simulink model "FHA_2P4S_Boosted"  (R2018a)
settings: Solver=VariableStepAuto  StartTime=0.0  StopTime=0.01  MaxStep=1e-5  RelTol=1e-3
values from neighbouring files (symbols this model uses):
  fop = 203    [inductance_calculation.m]
  M = 10^6*M    (= 4.12942555049)    [design_code.m]    (also in inductance_calculation.m = [M11 M12; M12' M22])
  R = [R11 R12;R12' R22]    [inductance_calculation.m]
  Vin_peak = 127    [inductance_calculation.m]
libraries: powerlib x49, powerlib_meascontrol x6
settings Model: Creator=user  LastModifiedBy=enes_

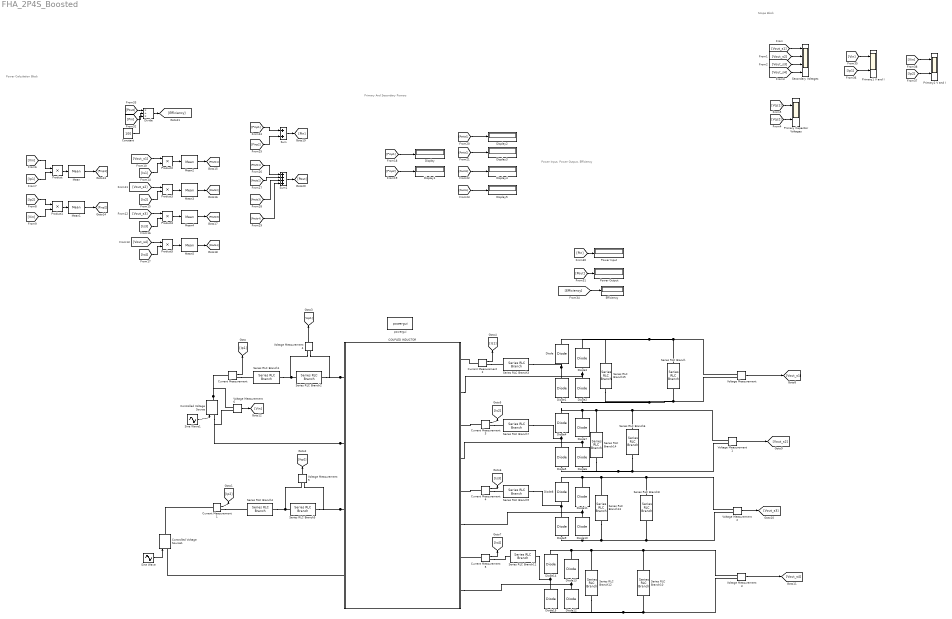
== system FHA_2P4S_Boosted ==
  note: Scope Block
  note: Primary And Secondary Powers
  note: Power Calculation Block
  note: Power Input,
      | Power Output,
      | Efficiency
  COUPLED INDUCTOR : Subsystem
  Constant : Constant  Value=100
  Controlled Voltage Source : powerlib/Electrical Sources/Controlled Voltage Source  Initialize=on  Source_Type=AC  Amplitude=0  Phase=0  Frequency=0  Measurements=None
  Controlled Voltage Source1 : powerlib/Electrical Sources/Controlled Voltage Source  Initialize=on  Source_Type=AC  Amplitude=0  Phase=0  Frequency=0  Measurements=None
  Current Measurement{,1..5} (6 alike) : powerlib/Measurements/Current Measurement  PhasorSimulation=off  OutputType=Complex  PSBequivalent=0
  Diode{,1..15} (16 alike) : powerlib/Power Electronics/Diode  Ron=0.001  Lon=0  Vf=0.8  IC=0  UseSnubber=0  Rs=inf  Cs=250e-9  Measurements=off
  Display{,1..5} (6 alike) : Display
  Divide : Product  Inputs=*/*
  Efficiency : Display
  Mean{,1..5} (6 alike) : powerlib_meascontrol/Measurements/Mean  Freq=fop*1000  Vinit=0  Ts=0
  Power Input : Display
  Power Output : Display
  Primary Capacitor Voltages : Scope  NumInputPorts=2
  Primary1 V and I : Scope  NumInputPorts=2
  Primary2 V and I : Scope  NumInputPorts=2
  Product{,1..5} (6 alike) : Product
  Secondary Voltages : Scope  NumInputPorts=4
  Series RLC Branch{,6,8,10} (4 alike) : powerlib/Elements/Series RLC Branch  LConnTagsString=__new0  RConnTagsString=__new0  BranchType=R  Resistance=15  Inductance=1e-3  SetiL0=off  InitialCurrent=0  Capacitance=1e-6  Setx0=off  InitialVoltage=0  Measurements=None
  Series RLC Branch1 : powerlib/Elements/Series RLC Branch  LConnTagsString=__new0  RConnTagsString=__new0  BranchType=R  Resistance=0.01  Inductance=1e-3  SetiL0=off  InitialCurrent=0  Capacitance=1e-6  Setx0=off  InitialVoltage=0  Measurements=None
  Series RLC Branch{3,7,9,11} (4 alike) : powerlib/Elements/Series RLC Branch  LConnTagsString=__new0  RConnTagsString=__new0  BranchType=C  Resistance=0.01  Inductance=1e-3  SetiL0=off  InitialCurrent=0  Capacitance=13.2e-9  Setx0=off  InitialVoltage=0  Measurements=None
  Series RLC Branch{12..15} (4 alike) : powerlib/Elements/Series RLC Branch  LConnTagsString=__new0  RConnTagsString=__new0  BranchType=C  Resistance=70  Inductance=1e-3  SetiL0=off  InitialCurrent=0  Capacitance=1e-6  Setx0=off  InitialVoltage=0  Measurements=None
  Series RLC Branch2 : powerlib/Elements/Series RLC Branch  LConnTagsString=__new0  RConnTagsString=__new0  BranchType=C  Resistance=0.01  Inductance=1e-3  SetiL0=off  InitialCurrent=0  Capacitance=8.4e-9  Setx0=off  InitialVoltage=0  Measurements=None
  Series RLC Branch4 : powerlib/Elements/Series RLC Branch  LConnTagsString=__new0  RConnTagsString=__new0  BranchType=R  Resistance=0.01  Inductance=1e-3  SetiL0=off  InitialCurrent=0  Capacitance=1e-6  Setx0=off  InitialVoltage=0  Measurements=None
  Series RLC Branch5 : powerlib/Elements/Series RLC Branch  LConnTagsString=__new0  RConnTagsString=__new0  BranchType=C  Resistance=0.01  Inductance=1e-3  SetiL0=off  InitialCurrent=0  Capacitance=8.4e-9  Setx0=off  InitialVoltage=0  Measurements=None
  Sine Wave : Sin  Amplitude=Vin_peak  Frequency=fop*1000*2*pi  SampleTime=0
  Sine Wave1 : Sin  Amplitude=Vin_peak  Frequency=fop*1000*2*pi  SampleTime=0
  Sum : Sum
  Sum1 : Sum  Inputs=++++
  Voltage Measurement{,1..6} (7 alike) : powerlib/Measurements/Voltage Measurement  PhasorSimulation=off  OutputType=Complex  PSBequivalent=0
  powergui : powerlib/powergui  Priority=1  SimulationMode=Continuous  SampleTime=50e-6  frequency=60  Iterations=50  frequencyindice=0  Pbase=100e6  ErrMax=1e-4  UnitsV=kV  UnitsW=MW  buscounter=0  FunctionMessages=off  echomessages=off  EnableUseOfTLC=off  CurrentSourceSwitches=off  DisableSnubberDevices=off  DisableRonSwitches=off  DisableVfSwitches=off  DisplayEquations=off  SolverType=Tustin/Backward Euler (TBE)  Interpol=off  ExternalGateDelay=off  methode=off  Ts=100  x0status=blocks  SPID=on  SwTol=0  HookPort=off  RestoreLinks=warning  ResistiveCurrentMeasurement=off  Frange=[0:2:500]  Ylog=off  Xlog=on  ShowGrid=off  save=off  variable=ZData  structure=0  ZoomFFT=off  StartTime=0.0  cycles=1  DisplayStyle=1  fundamental=60  FreqAxis=off  MaxFrequency=1000  frequencyindicesteady=1  RmsSteady=1  display=off
  wires:
  Divide/1 -> [Efficiency]
  [Ip1] -> Primary1 V and I/2
  [Efficiency] -> Efficiency/1
  [Pouts4] -> Sum1/4
  [Vin] -> Primary1 V and I/1
  [Vin] -> Primary2 V and I/1
  Voltage Measurement2/1 -> [Vout_s3]
  [Pin] -> Power Input/1
  Mean1/1 -> [Pinp2]
  [Pin] -> Divide/2
  [Pout] -> Divide/1
  [Vout_s2] -> Product3/1
  Constant/1 -> Divide/3
  Current Measurement/1 -> [Ip1]
  [Pouts3] -> Sum1/3
  [Pinp1] -> Sum/1
  [Pout] -> Power Output/1
  [Vout_s3] -> Secondary Voltages/3
  [Vout_s1] -> Product2/1
  Current Measurement4/1 -> [Is3]
  [Pouts2] -> Sum1/2
  Sum1/1 -> [Pout]
  Current Measurement1/1 -> [Ip2]
  [Is2] -> Product3/2
  [Pouts2] -> Display3/1
  [Pouts3] -> Display4/1
  [Pinp2] -> Display1/1
  [Pouts1] -> Display2/1
  [Pinp2] -> Sum/2
  [Vcp1] -> Primary Capacitor Voltages/1
  [Pinp1] -> Display/1
  [Pouts4] -> Display5/1
  Product5/1 -> Mean5/1
  [Vin] -> Product/1
  [Vout_s2] -> Secondary Voltages/2
  Mean/1 -> [Pinp1]
  [Is4] -> Product5/2
  Mean4/1 -> [Pouts3]
  Mean2/1 -> [Pouts1]
  Product2/1 -> Mean2/1
  Product4/1 -> Mean4/1
  [Vcp2] -> Primary Capacitor Voltages/2
  [Vout_s4] -> Product5/1
  [Is1] -> Product2/2
  [Vin] -> Product1/2
  [Vout_s1] -> Secondary Voltages/1
  Voltage Measurement3/1 -> [Vout_s4]
  [Ip1] -> Product/2
  [Pouts1] -> Sum1/1
  Voltage Measurement4/1 -> [Vcp1]
  [Vout_s3] -> Product4/1
  Voltage Measurement1/1 -> [Vout_s2]
  Sine Wave1/1 -> Controlled Voltage Source/1
  Current Measurement3/1 -> [Is2]
  Product1/1 -> Mean1/1
  Mean3/1 -> [Pouts2]
  Sum/1 -> [Pin]
  [Ip2] -> Product1/1
  Mean5/1 -> [Pouts4]
  Voltage Measurement/1 -> [Vout_s1]
  [Vout_s4] -> Secondary Voltages/4
  Sine Wave/1 -> Controlled Voltage Source1/1
  [Ip2] -> Primary2 V and I/2
  [Is3] -> Product4/2
  Current Measurement2/1 -> [Is1]
  Product/1 -> Mean/1
  Voltage Measurement5/1 -> [Vcp2]
  Product3/1 -> Mean3/1
  Current Measurement5/1 -> [Is4]
  Voltage Measurement6/1 -> [Vin]
  connections:
  Diode14/RConn1 -- Diode13/RConn1 -- Series RLC Branch12/LConn1 -- Series RLC Branch10/LConn1 -- Voltage Measurement3/LConn1
  Series RLC Branch2/LConn1 -- Series RLC Branch1/LConn1 -- Voltage Measurement4/LConn1
  Series RLC Branch5/LConn1 -- Series RLC Branch4/LConn1 -- Voltage Measurement5/LConn1
  Diode4/RConn1 -- Series RLC Branch14/LConn1 -- Voltage Measurement1/LConn1 -- Series RLC Branch6/LConn1 -- Diode7/RConn1
  Diode9/LConn1 -- Series RLC Branch13/RConn1 -- Voltage Measurement2/LConn2 -- Series RLC Branch8/RConn1 -- Diode10/LConn1
  Controlled Voltage Source/RConn1 -- Current Measurement/LConn1 -- Voltage Measurement6/LConn1
  COUPLED INDUCTOR/RConn3 -- Series RLC Branch5/RConn1 -- Voltage Measurement5/LConn2
  COUPLED INDUCTOR/RConn1 -- Series RLC Branch2/RConn1 -- Voltage Measurement4/LConn2
  Diode8/RConn1 -- Diode11/RConn1 -- Series RLC Branch13/LConn1 -- Series RLC Branch8/LConn1 -- Voltage Measurement2/LConn1
  COUPLED INDUCTOR/RConn2 -- Controlled Voltage Source/LConn1 -- Voltage Measurement6/LConn2
  Current Measurement1/LConn1 -- Controlled Voltage Source1/RConn1
  Current Measurement/RConn1 -- Series RLC Branch1/RConn1
  Current Measurement3/RConn1 -- Series RLC Branch7/LConn1
  Current Measurement4/LConn1 -- COUPLED INDUCTOR/LConn5
  Current Measurement5/RConn1 -- Series RLC Branch11/LConn1
  Current Measurement2/LConn1 -- COUPLED INDUCTOR/LConn1
  Current Measurement5/LConn1 -- COUPLED INDUCTOR/LConn7
  Current Measurement2/RConn1 -- Series RLC Branch3/LConn1
  COUPLED INDUCTOR/RConn4 -- Controlled Voltage Source1/LConn1
  Current Measurement3/LConn1 -- COUPLED INDUCTOR/LConn3
  Current Measurement4/RConn1 -- Series RLC Branch9/LConn1
  Current Measurement1/RConn1 -- Series RLC Branch4/RConn1
  Diode1/RConn1 -- Series RLC Branch3/RConn1 -- Diode/LConn1
  Diode3/LConn1 -- COUPLED INDUCTOR/LConn2 -- Diode2/RConn1
  Voltage Measurement/LConn1 -- Diode3/RConn1 -- Diode/RConn1 -- Series RLC Branch15/LConn1 -- Series RLC Branch/LConn1
  Voltage Measurement/LConn2 -- Diode2/LConn1 -- Diode1/LConn1 -- Series RLC Branch15/RConn1 -- Series RLC Branch/RConn1
  Series RLC Branch6/RConn1 -- Diode6/LConn1 -- Diode5/LConn1 -- Series RLC Branch14/RConn1 -- Voltage Measurement1/LConn2
  Diode7/LConn1 -- COUPLED INDUCTOR/LConn4 -- Diode6/RConn1
  Diode5/RConn1 -- Series RLC Branch7/RConn1 -- Diode4/LConn1
  Diode9/RConn1 -- Series RLC Branch9/RConn1 -- Diode8/LConn1
  Diode11/LConn1 -- COUPLED INDUCTOR/LConn6 -- Diode10/RConn1
  Voltage Measurement3/LConn2 -- Series RLC Branch12/RConn1 -- Diode12/LConn1 -- Diode15/LConn1 -- Series RLC Branch10/RConn1
  Diode13/LConn1 -- COUPLED INDUCTOR/LConn8 -- Diode12/RConn1
  Diode15/RConn1 -- Series RLC Branch11/RConn1 -- Diode14/LConn1

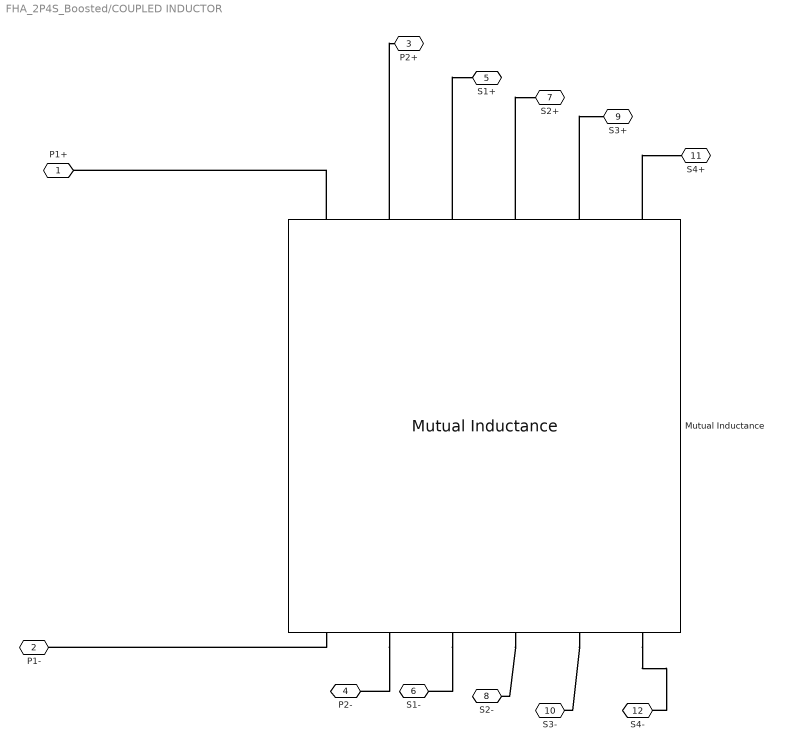
== system FHA_2P4S_Boosted/COUPLED INDUCTOR ==
  Mutual Inductance : powerlib/Elements/Mutual Inductance  LConnTagsString=a|b|c|L4|L5|L6  RConnTagsString=A|B|C|R4|R5|R6  TypeOfMutual=Generalized mutual inductance  NumberOfWindings=6  SelfImpedance1=[1.1 1.1e-03]  SelfImpedance2=[ 1.1 1.1e-03]  ThreeWindings=on  SelfImpedance3=[ 1.1 1.1e-03]  MutualImpedance=[1.0 1.0e-03]  InductanceMatrix=M * 1e-6  ResistanceMatrix=R*0.001  Measurements=None
      settings: AttributesFormatString=\n  SourceProductName=Simscape Power Systems  SourceProductBaseCode=PS
  P1+ : PMIOPort  Side=Right
  P1- : PMIOPort  Port=2  Side=Right
  P2+ : PMIOPort  Port=3  Side=Right
  P2- : PMIOPort  Port=4  Side=Right
  S1+ : PMIOPort  Port=5  Side=Left
  S1- : PMIOPort  Port=6  Side=Left
  S2+ : PMIOPort  Port=7  Side=Left
  S2- : PMIOPort  Port=8  Side=Left
  S3+ : PMIOPort  Port=9  Side=Left
  S3- : PMIOPort  Port=10  Side=Left
  S4+ : PMIOPort  Port=11  Side=Left
  S4- : PMIOPort  Port=12  Side=Left
  connections:
  Mutual Inductance/LConn2 -- P2-/RConn1
  Mutual Inductance/LConn5 -- S3-/RConn1
  Mutual Inductance/RConn5 -- S3+/RConn1
  Mutual Inductance/RConn4 -- S2+/RConn1
  Mutual Inductance/LConn6 -- S4-/RConn1
  Mutual Inductance/RConn1 -- P1+/RConn1
  Mutual Inductance/LConn1 -- P1-/RConn1
  Mutual Inductance/RConn2 -- P2+/RConn1
  Mutual Inductance/LConn4 -- S2-/RConn1
  Mutual Inductance/LConn3 -- S1-/RConn1
  Mutual Inductance/RConn3 -- S1+/RConn1
  Mutual Inductance/RConn6 -- S4+/RConn1
